simulink model "Introduction_to_Simulink"  (R2021a)
settings: Solver=VariableStepAuto  StartTime=0.0  StopTime=10.0  MaxStep=1e-3  RelTol=1e-3
settings Model: Creator=HP  LastModifiedBy=HP

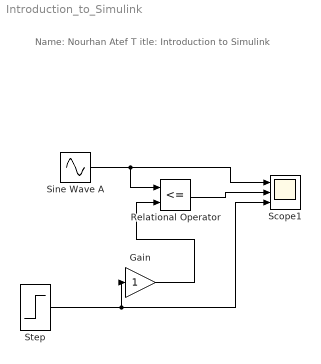
== system Introduction_to_Simulink ==
  note: Name: Nourhan Atef
      |
      | T itle: Introduction to Simulink
  Gain : Gain
  Relational Operator : RelationalOperator  Operator=<=  OutDataTypeStr=boolean  RndMeth=Simplest
  Scope1 : Scope  NumInputPorts=3
  Sine Wave A : Sin  Frequency=2*pi*1  SampleTime=0
  Step : Step  Time=2  SampleTime=0
  wires:
  Relational Operator/1 -> Scope1/2
  Sine Wave A/1 -> Scope1/1, Relational Operator/1
  Step/1 -> Gain/1, Scope1/3
  Gain/1 -> Relational Operator/2
